simulink model "IdealGen_load_abc"  (R2023b)
settings: Solver=VariableStepAuto  StartTime=0.0  StopTime=Tend  RelTol=1e-3
undefined symbols (not defined in the file): C_hv_km, Cagg, f_nom, Ibase_hv, Ibase_lv, L_comp, L_grid, L_hv_km, l_t_ehvhv, l_t_hvmv, l_t_mvlv, Lagg, nWT, phase_shift_test_state, phase_shifts, PnomWT, R_grid, R_hv_km, r_t_ehvhv, r_t_hvmv, r_t_mvlv, Ragg, rocof_slope, Rocof_test_state, Sbase1, Sbase_t1, Trocof_end, Trocof_start, Ts_power, Vbase_ehv, Vbase_hv, Vbase_lv, Vbase_mv, voltage_sag_test_state
libraries: spsThreePhasePISectionLineLib x11, spsPower3phInstantaneousLib x5, spsControlledVoltageSourceLib x3, spsGroundLib x3, spsThreePhaseVIMeasurementLib x3, spsThreePhaseSeriesRLCBranchLib x3, spsThreePhaseTransformerTwoWindingsLib x3, spsdq0toabcLib x1, simulink x1, spsSampleandHoldLib x1, spsMultimeterLib x1, spsThreePhaseSeriesRLCLoadLib x1
settings Model: Creator=s183702  LastModifiedBy=Martin Pedersen

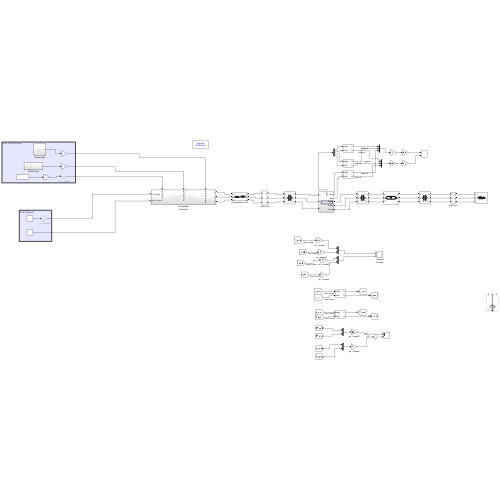
[thumbnail: Simulink's stored preview of the top-level diagram]
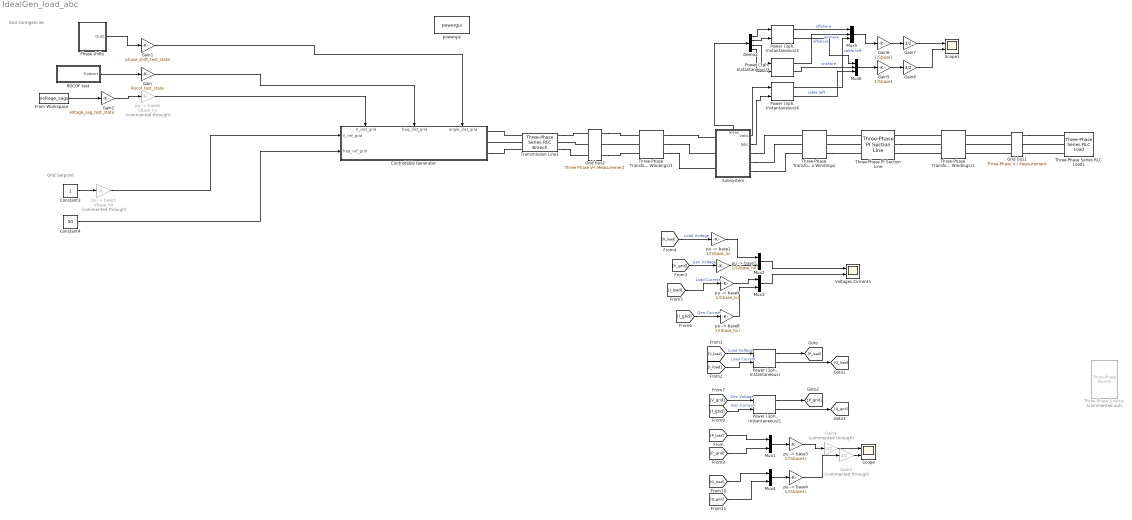
== system IdealGen_load_abc ==
  note: Grid Contigencies
  note: Grid Setpoint
  Constant3 : Constant
  Constant4 : Constant  Value=50
  Controllable Generator : Subsystem
      settings: PortSchema="{\"entries\":[{\"content\":{\"sides\":[{\"content\":{\"connectorIds\":[\"In1\",\"In2\"]},\"type\":\"ConnectorPlacement.EquallySpacedRectSide\",\"uuid\":\"c82e3ee4-47de-4631-9682-a189e406d2fd\"},{\"content\":{\"connectorIds\":[\"RConn1\",\"RConn2\",\"RConn3\"],\"side\":\"RIGHT\"},\"type\":\"ConnectorPlacement.EquallySpacedRectSide\",\"uuid\":\"b806e225-811d-4112-8c3d-45e9b8086e84\"},{\"content\":{\"connectorIds\":[\"In3\",\"In4\",\"In5\"],\"side\":\"TOP\"},\"type\":\"ConnectorPlacement.EquallySpacedRectSide\",\"uuid\":\"c79b677b-bc74-4454-b0f0-10f0f27e0767\"}]},\"type\":\"ConnectorPlacement.EquallySpacedConnector\",\"uuid\":\"44354c03-b4f0-403a-803b-b669dc1296a6\"}],\"packageUris\":[\"http://schema.mathworks.com/mf0/Connector/R2020b\"],\"version\":\"1.0\"}"
  Demux : Demux
  From Workspace : FromWorkspace  VariableName=voltage_sags
  Gain : Gain  Gain=Rocof_test_state
  Gain1 : Gain  Gain=phase_shift_test_state
  Gain2 : Gain  Gain=voltage_sag_test_state
  Gain3 : Gain  Commented=through  Gain=3/2
  Gain4 : Gain  Commented=through  Gain=3/2
  Gain5 : Gain  Gain=1/Sbase1
  Gain6 : Gain  Gain=1/Sbase1
  Gain7 : Gain  Gain=3/2
  Gain8 : Gain  Gain=3/2
  Grid bus1 : spsThreePhaseVIMeasurementLib/Three-Phase V-I Measurement  VoltageMeasurement=phase-to-phase  SetLabelV=on  LabelV=V_load  Vpu=off  VpuLL=off  CurrentMeasurement=yes  SetLabelI=on  LabelI=I_load  Ipu=off  Pbase=100e6  Vbase=500e3  OutputType=Complex  PhasorSimulation=off  PSBequivalent=0
  Grid bus2 : spsThreePhaseVIMeasurementLib/Three-Phase V-I Measurement  VoltageMeasurement=phase-to-phase  SetLabelV=on  LabelV=V_grid  Vpu=off  VpuLL=off  CurrentMeasurement=yes  SetLabelI=on  LabelI=I_grid  Ipu=off  Pbase=100e6  Vbase=500e3  OutputType=Complex  PhasorSimulation=off  PSBequivalent=0
  Mux{1..4} (4 alike) : Mux  Inputs=2
  Mux5 : Mux  Inputs=3
  Mux6 : Mux  Inputs=3
  Phase shifts : Subsystem
  Power (3ph, Instantaneous){,1..4} (5 alike) : spsPower3phInstantaneousLib/Power (3ph, Instantaneous)
  ROCOF test : Subsystem
  Scope : Scope  NumInputPorts=2
  Scope1 : Scope  NumInputPorts=2
  Subsystem : Subsystem
      settings: PortSchema="{\"entries\":[{\"content\":{\"sides\":[{\"content\":{\"connectorIds\":[\"LConn1\",\"LConn2\",\"LConn3\"]},\"type\":\"ConnectorPlacement.EquallySpacedRectSide\",\"uuid\":\"1e75b8ae-1ae2-41d3-b362-6bec791dcf00\"},{\"content\":{\"connectorIds\":[\"Out1\",\"Out2\",\"RConn1\",\"RConn2\",\"RConn3\"],\"side\":\"RIGHT\"},\"type\":\"ConnectorPlacement.EquallySpacedRectSide\",\"uuid\":\"b9649e6f-c713-4552-95ab-bed4ae3fc4ed\"},{\"content\":{\"connectorIds\":[\"Out3\"],\"side\":\"TOP\"},\"type\":\"ConnectorPlacement.EquallySpacedRectSide\",\"uuid\":\"245e241a-8feb-4dbf-8b97-336629a28915\"}]},\"type\":\"ConnectorPlacement.EquallySpacedConnector\",\"uuid\":\"8d181cc9-19cf-4cb2-b946-858b4ed04b70\"}],\"packageUris\":[\"http://schema.mathworks.com/mf0/Connector/R2020b\"],\"version\":\"1.0\"}"
  Three-Phase PI Section Line : spsThreePhasePISectionLineLib/Three-Phase PI Section Line  LConnTagsString=a|b|c  RConnTagsString=A|B|C  Length=1  Frequency=50  Resistances=[ 1 3]*Ragg  Inductances=[ 1 3]*Lagg  Capacitances=[ 1 0.6]*Cagg
  Three-Phase Series RLC Load1 : spsThreePhaseSeriesRLCLoadLib/Three-Phase Series RLC Load  LConnTagsString=A|B|C  Configuration=Y (grounded)  NominalVoltage=Vbase_lv*sqrt(3/2)  Vabc=[1e3 1e3 1e3]  Vabcp=[1e3 1e3 1e3]  NominalFrequency=f_nom  UnbalancedPower=off  ActivePower=PnomWT*nWT  InductivePower=0  CapacitivePower=0  Pabc=[10e3 9e3 11e3]  QLabc=[100 90 110]  QCabc=[100 90 110]  Pabcp=[10e3 9e3 11e3]  QLabcp=[100 90 110]  QCabcp=[100 90 110]  Measurements=None  LoadType=constant PQ
  Three-Phase Transformer (Two Windings) : spsThreePhaseTransformerTwoWindingsLib/Three-Phase Transformer (Two Windings)  Winding1Connection=Yg  Winding2Connection=Yg  CoreType=Three single-phase transformers  SetSaturation=off  Hysteresis=off  DataFile='hysteresis'  SetInitialFlux=off  Measurements=None  UNITS=pu  NominalPower=[ Sbase1 , f_nom ]  Winding1=[ Vbase_hv*sqrt(3/2) , r_t_hvmv/2 , l_t_hvmv/2]  Winding2=[ Vbase_mv*sqrt(3/2) , r_t_hvmv/2, l_t_hvmv/2 ]  Rm=500  Lm=500  L0=0.5  Saturation=[ 0,0 ; 0.0024,1.2 ; 1.0,1.52 ]  InitialFluxes=[ 0.8 , -0.8 , 0.7 ]  BreakLoop=off  DiscreteSolver=Trapezoidal iterative  DataType=off  TransfoNumber=1
  Three-Phase Transformer (Two Windings)1 : spsThreePhaseTransformerTwoWindingsLib/Three-Phase Transformer (Two Windings)  Winding1Connection=Yg  Winding2Connection=Yg  CoreType=Three single-phase transformers  SetSaturation=off  Hysteresis=off  DataFile='hysteresis'  SetInitialFlux=off  Measurements=None  UNITS=pu  NominalPower=[ Sbase_t1 , f_nom ]  Winding1=[ Vbase_mv*sqrt(3/2) , r_t_mvlv/2 , l_t_mvlv/2]  Winding2=[ Vbase_lv*sqrt(3/2) , r_t_mvlv/2, l_t_mvlv/2 ]  Rm=500  Lm=500  L0=0.5  Saturation=[ 0,0 ; 0.0024,1.2 ; 1.0,1.52 ]  InitialFluxes=[ 0.8 , -0.8 , 0.7 ]  BreakLoop=off  DiscreteSolver=Trapezoidal iterative  DataType=off  TransfoNumber=1
  Three-Phase Transformer (Two Windings)3 : spsThreePhaseTransformerTwoWindingsLib/Three-Phase Transformer (Two Windings)  Winding1Connection=Yg  Winding2Connection=Yg  CoreType=Three single-phase transformers  SetSaturation=off  Hysteresis=off  DataFile='hysteresis'  SetInitialFlux=off  Measurements=None  UNITS=pu  NominalPower=[ Sbase1*1.05, f_nom ]  Winding1=[ Vbase_ehv*sqrt(3/2) , r_t_ehvhv/2 , l_t_ehvhv/2]  Winding2=[ Vbase_hv*sqrt(3/2) ,r_t_ehvhv/2 , l_t_ehvhv/2 ]  Rm=500  Lm=500  L0=0.5  Saturation=[ 0,0 ; 0.0024,1.2 ; 1.0,1.52 ]  InitialFluxes=[ 0.8 , -0.8 , 0.7 ]  BreakLoop=off  DiscreteSolver=Trapezoidal iterative  DataType=off  TransfoNumber=1
  Three-Phase Source : spsThreePhaseSourceLib/Three-Phase Source  Commented=on  InternalConnection=Yg  VoltagePhases=off  Voltage=0.8*Vbase_lv*sqrt(3)/sqrt(2)  PhaseAngle=0  Voltage_phases=[25e3 25e3 25e3]/sqrt(3)  PhaseAngles_phases=[0 -120 +120]  Frequency=50  NonIdealSource=off  SpecifyImpedance=off  Resistance=0.8929  Inductance=16.58e-3  ShortCircuitLevel=100e6  BaseVoltage=25e3  XRratio=7  BusType=swing  Pref=10e3  Qref=0  Prefabc=[10e3, 10e3, 10e3]  Qrefabc=[0, 0, 0]  Qmin=-inf  Qmax=inf
  Transmission Line1 : spsThreePhaseSeriesRLCBranchLib/Three-Phase Series RLC Branch  LConnTagsString=A|B|C  RConnTagsString=A|B|C  BranchType=RL  Resistance=R_grid  Inductance=L_grid  Capacitance=0  Measurements=None
  Voltages Currents : Scope  NumInputPorts=2
  powergui : spspowerguiLib/powergui  Priority=1  SimulationMode=Discrete  SampleTime=Ts_power  frequency=60  Iterations=50  frequencyindice=50  Pbase=100e6  ErrMax=1e-4  UnitsV=kV  UnitsW=MW  buscounter=0  FunctionMessages=off  echomessages=off  EnableUseOfTLC=off  CurrentSourceSwitches=off  DisableSnubberDevices=off  DisableRonSwitches=off  DisableVfSwitches=off  DisplayEquations=off  AutomaticDiscreteSolvers=off  SolverType=Tustin/Backward Euler (TBE)  Interpol=off  ExternalGateDelay=off  methode=off  Ts=100  x0status=blocks  SPID=on  SwTol=0  HookPort=off  NonlinearTolerance=1e-4  nMaxIteration=100  ContinueOnMaxIteration=off  RestoreLinks=warning  ResistiveCurrentMeasurement=off  Frange=[0:2:500]  Ylog=off  Xlog=on  ShowGrid=off  save=off  variable=ZData  structure=0  ZoomFFT=off  StartTime=0.0  cycles=1  DisplayStyle=1  fundamental=60  FreqAxis=off  MaxFrequency=1000  frequencyindicesteady=1  RmsSteady=1  display=off
  "pu -> base1" : Gain  Gain=1/(Vbase_lv)
  "pu -> base3" : Gain  Gain=1/(Sbase1)
  "pu -> base4" : Gain  Gain=1/(Sbase1)
  "pu -> base5" : Gain  Commented=through  Gain=Vbase_hv
  "pu -> base6" : Gain  Commented=through  Gain=Vbase_hv
  "pu -> base7" : Gain  Gain=1/(Vbase_hv)
  "pu -> base8" : Gain  Gain=1/(Ibase_hv)
  "pu -> base9" : Gain  Gain=1/(Ibase_lv)
  wires:
  [I_load] -> "pu -> base9"/1  "Load Current"
  [V_load] -> "pu -> base1"/1  "Load Voltage"
  [V_grid] -> "pu -> base7"/1  "Gen Voltage"
  [I_grid] -> "pu -> base8"/1  "Gen Current"
  Mux3/1 -> Voltages Currents/2
  "pu -> base5"/1 -> Controllable Generator/1(V_ref_grid)
  Constant4/1 -> Controllable Generator/2(freq_ref_grid)
  Gain/1 -> Controllable Generator/4(freq_dist_grid)
  Gain1/1 -> Controllable Generator/5(angle_dist_grid)
  [V_load] -> "Power (3ph, Instantaneous)"/1  "Load Voltage"
  [I_load] -> "Power (3ph, Instantaneous)"/2  "Load Current"
  [V_grid] -> "Power (3ph, Instantaneous)1"/1  "Gen Voltage"
  [I_grid] -> "Power (3ph, Instantaneous)1"/2  "Gen Current"
  "Power (3ph, Instantaneous)"/1 -> [P_load]
  "Power (3ph, Instantaneous)"/2 -> [Q_load]
  "Power (3ph, Instantaneous)1"/1 -> [P_grid]
  "Power (3ph, Instantaneous)1"/2 -> [Q_grid]
  [Q_load] -> Mux4/1
  [Q_grid] -> Mux4/2
  [P_grid] -> Mux1/2
  [P_load] -> Mux1/1
  Mux4/1 -> "pu -> base4"/1
  Mux1/1 -> "pu -> base3"/1
  "pu -> base3"/1 -> Gain4/1
  "pu -> base4"/1 -> Gain3/1
  Constant3/1 -> "pu -> base5"/1
  Phase shifts/1(Out2) -> Gain1/1
  From Workspace/1 -> Gain2/1
  ROCOF test/1(Outport) -> Gain/1
  "pu -> base6"/1 -> Controllable Generator/3(V_dist_grid)
  Gain2/1 -> "pu -> base6"/1
  Mux2/1 -> Voltages Currents/1
  "pu -> base1"/1 -> Mux2/1
  "pu -> base7"/1 -> Mux2/2
  "pu -> base8"/1 -> Mux3/2
  "pu -> base9"/1 -> Mux3/1
  Gain3/1 -> Scope/2
  Gain4/1 -> Scope/1
  "Power (3ph, Instantaneous)3"/1 -> Mux5/2  "onshore"
  Demux/3 -> "Power (3ph, Instantaneous)3"/1
  Demux/2 -> "Power (3ph, Instantaneous)2"/2
  Subsystem/3(meas) -> Demux/1
  "Power (3ph, Instantaneous)2"/1 -> Mux5/1  "offshore"
  "Power (3ph, Instantaneous)3"/2 -> Mux6/2  "onshore"
  Demux/4 -> "Power (3ph, Instantaneous)3"/2
  "Power (3ph, Instantaneous)2"/2 -> Mux6/1  "offshore"
  Demux/1 -> "Power (3ph, Instantaneous)2"/1
  "Power (3ph, Instantaneous)4"/1 -> Mux5/3  "cable left"
  "Power (3ph, Instantaneous)4"/2 -> Mux6/3  "cable left"
  Mux5/1 -> Gain6/1
  Mux6/1 -> Gain5/1
  Gain6/1 -> Gain7/1
  Gain5/1 -> Gain8/1
  Gain7/1 -> Scope1/1
  Gain8/1 -> Scope1/2
  Subsystem/1(Vabc) -> "Power (3ph, Instantaneous)4"/1
  Subsystem/2(Iabc) -> "Power (3ph, Instantaneous)4"/2
  connections:
  Three-Phase Transformer (Two Windings)1/LConn1 -- Three-Phase PI Section Line/RConn1
  Grid bus1/RConn1 -- Three-Phase Series RLC Load1/LConn1
  Three-Phase Series RLC Load1/LConn2 -- Grid bus1/RConn2
  Grid bus1/RConn3 -- Three-Phase Series RLC Load1/LConn3
  Transmission Line1/RConn1 -- Grid bus2/LConn1
  Grid bus2/LConn2 -- Transmission Line1/RConn2
  Transmission Line1/RConn3 -- Grid bus2/LConn3
  Transmission Line1/LConn1 -- Controllable Generator/RConn1
  Transmission Line1/LConn2 -- Controllable Generator/RConn2
  Controllable Generator/RConn3 -- Transmission Line1/LConn3
  Three-Phase PI Section Line/LConn2 -- Three-Phase Transformer (Two Windings)/RConn2
  Three-Phase PI Section Line/LConn1 -- Three-Phase Transformer (Two Windings)/RConn1
  Three-Phase Transformer (Two Windings)/RConn3 -- Three-Phase PI Section Line/LConn3
  Three-Phase PI Section Line/RConn2 -- Three-Phase Transformer (Two Windings)1/LConn2
  Three-Phase Transformer (Two Windings)1/LConn3 -- Three-Phase PI Section Line/RConn3
  Grid bus1/LConn1 -- Three-Phase Transformer (Two Windings)1/RConn1
  Grid bus1/LConn2 -- Three-Phase Transformer (Two Windings)1/RConn2
  Grid bus1/LConn3 -- Three-Phase Transformer (Two Windings)1/RConn3
  Three-Phase Transformer (Two Windings)3/LConn2 -- Grid bus2/RConn2
  Grid bus2/RConn1 -- Three-Phase Transformer (Two Windings)3/LConn1
  Grid bus2/RConn3 -- Three-Phase Transformer (Two Windings)3/LConn3
  Three-Phase Transformer (Two Windings)3/RConn1 -- Subsystem/LConn1
  Subsystem/RConn1 -- Three-Phase Transformer (Two Windings)/LConn1
  Three-Phase Transformer (Two Windings)3/RConn2 -- Subsystem/LConn2
  Subsystem/RConn2 -- Three-Phase Transformer (Two Windings)/LConn2
  Three-Phase Transformer (Two Windings)3/RConn3 -- Subsystem/LConn3
  Subsystem/RConn3 -- Three-Phase Transformer (Two Windings)/LConn3

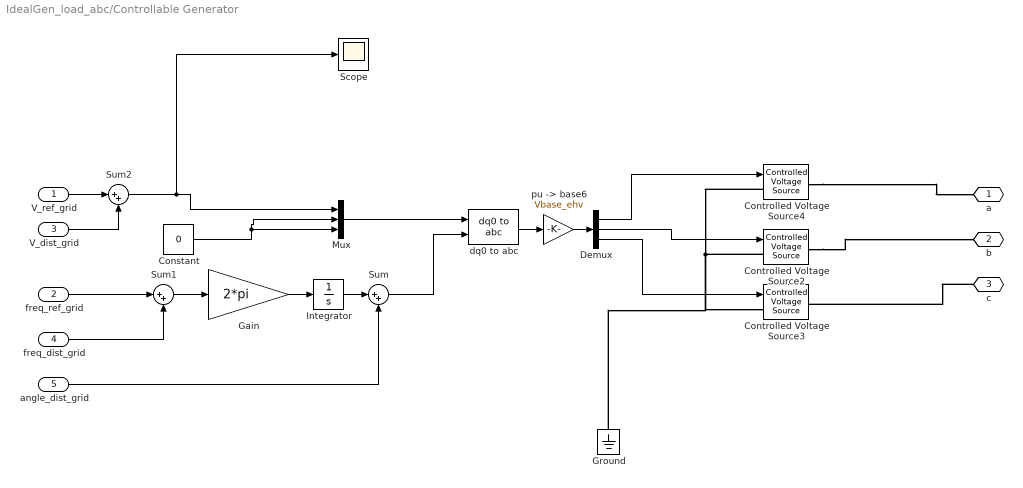
== system IdealGen_load_abc/Controllable Generator ==
  V_ref_grid : Inport
  freq_ref_grid : Inport  Port=2
  V_dist_grid : Inport  Port=3
  freq_dist_grid : Inport  Port=4
  angle_dist_grid : Inport  Port=5
  Constant : Constant  Value=0
  Controlled Voltage Source2 : spsControlledVoltageSourceLib/Controlled Voltage Source  Initialize=on  Source_Type=AC  Amplitude=Vbase_hv  Phase=-120  Frequency=50  Measurements=None
  Controlled Voltage Source3 : spsControlledVoltageSourceLib/Controlled Voltage Source  Initialize=on  Source_Type=AC  Amplitude=Vbase_hv  Phase=120  Frequency=50  Measurements=None
  Controlled Voltage Source4 : spsControlledVoltageSourceLib/Controlled Voltage Source  Initialize=on  Source_Type=AC  Amplitude=Vbase_hv  Phase=0  Frequency=50  Measurements=None
  Demux : Demux  Outputs=3
  Gain : Gain  Gain=2*pi
  Ground : spsGroundLib/Ground  LConnTagsString=a
  Integrator : Integrator
  Mux : Mux  Inputs=3
  Scope : Scope
  Sum : Sum  Inputs=|++
  Sum1 : Sum  Inputs=|++
  Sum2 : Sum  Inputs=|++
  dq0 to abc : spsdq0toabcLib/dq0 to abc  Alignment=90 degrees behind phase A axis
  "pu -> base6" : Gain  Gain=Vbase_ehv
  a : PMIOPort  Side=Right
  b : PMIOPort  Port=2  Side=Right
  c : PMIOPort  Port=3  Side=Right
  wires:
  Demux/1 -> Controlled Voltage Source4/1
  Demux/2 -> Controlled Voltage Source2/1
  Demux/3 -> Controlled Voltage Source3/1
  Mux/1 -> dq0 to abc/1
  Constant/1 -> Mux/2, Mux/3
  dq0 to abc/1 -> "pu -> base6"/1
  Sum2/1 -> Scope/1, Mux/1
  Gain/1 -> Integrator/1
  Integrator/1 -> Sum/1
  angle_dist_grid/1 -> Sum/2
  freq_dist_grid/1 -> Sum1/2
  Sum1/1 -> Gain/1
  freq_ref_grid/1 -> Sum1/1
  Sum/1 -> dq0 to abc/2
  V_ref_grid/1 -> Sum2/1
  V_dist_grid/1 -> Sum2/2
  "pu -> base6"/1 -> Demux/1
  connections:
  Controlled Voltage Source2/LConn1 -- Controlled Voltage Source4/LConn1 -- Ground/LConn1 -- Controlled Voltage Source3/LConn1
  c/RConn1 -- Controlled Voltage Source3/RConn1
  Controlled Voltage Source4/RConn1 -- a/RConn1
  Controlled Voltage Source2/RConn1 -- b/RConn1

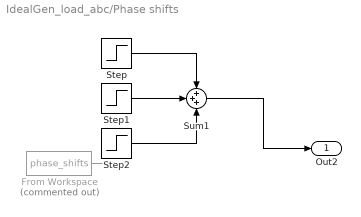
== system IdealGen_load_abc/Phase shifts ==
  From Workspace : FromWorkspace  Commented=on  VariableName=phase_shifts  OutputAfterFinalValue=Setting to zero
  Step : Step  Time=phase_shifts(1,1)  After=phase_shifts(1,2)  SampleTime=0
  Step1 : Step  Time=phase_shifts(2,1)  After=phase_shifts(2,2)  SampleTime=0
  Step2 : Step  Time=phase_shifts(3,1)  After=phase_shifts(3,2)  SampleTime=0
  Sum1 : Sum  Inputs=+++
  Out2 : Outport
  wires:
  Sum1/1 -> Out2/1
  Step/1 -> Sum1/1
  Step2/1 -> Sum1/3
  From Workspace/1 -> ?
  Step1/1 -> Sum1/2

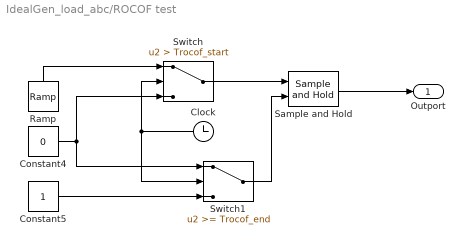
== system IdealGen_load_abc/ROCOF test ==
  Clock : Clock
  Constant4 : Constant  Value=0
  Constant5 : Constant
  Ramp : simulink/Sources/Ramp  slope=rocof_slope  start=Trocof_start  InitialOutput=0
  Sample and Hold : spsSampleandHoldLib/Sample and Hold  ic=0  Ts=0
      settings: LibrarySourceBlock=|
      | sps_lib/Control/Sample and
      | Hold
  Switch : Switch  Criteria=u2 > Threshold  Threshold=Trocof_start  SaturateOnIntegerOverflow=off  InputSameDT=off
  Switch1 : Switch  Threshold=Trocof_end  SaturateOnIntegerOverflow=off  InputSameDT=off
  Outport : Outport
  wires:
  Clock/1 -> Switch/2, Switch1/2
  Constant4/1 -> Switch/3, Switch1/1
  Sample and Hold/1 -> Outport/1
  Ramp/1 -> Switch/1
  Constant5/1 -> Switch1/3
  Switch/1 -> Sample and Hold/1
  Switch1/1 -> Sample and Hold/2

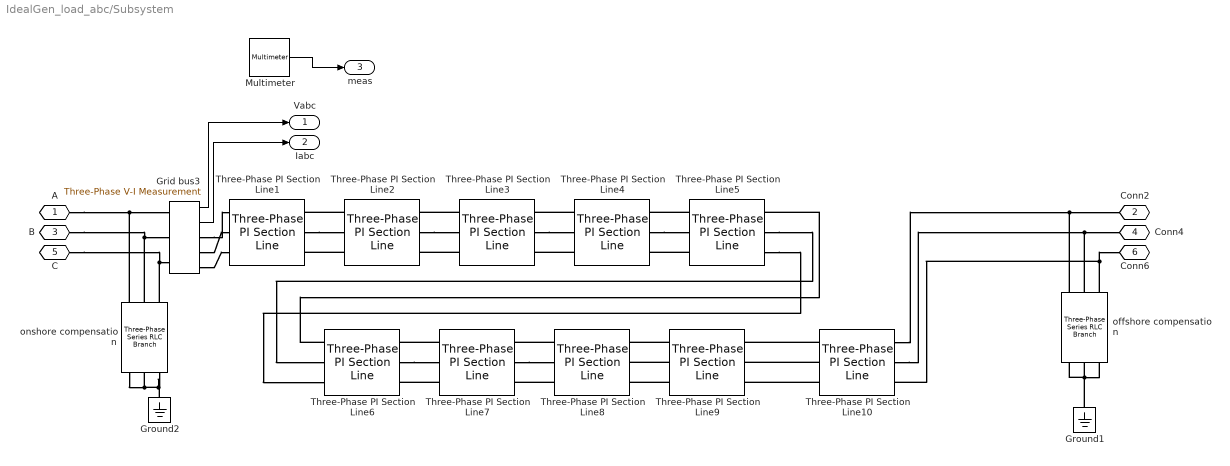
== system IdealGen_load_abc/Subsystem ==
  Grid bus3 : spsThreePhaseVIMeasurementLib/Three-Phase V-I Measurement  VoltageMeasurement=phase-to-ground  SetLabelV=off  LabelV=V_grid  Vpu=off  VpuLL=off  CurrentMeasurement=yes  SetLabelI=off  LabelI=I_grid  Ipu=off  Pbase=100e6  Vbase=500e3  OutputType=Complex  PhasorSimulation=off  PSBequivalent=0
  Ground1 : spsGroundLib/Ground  LConnTagsString=a
  Ground2 : spsGroundLib/Ground  LConnTagsString=a
  Multimeter : spsMultimeterLib/Multimeter  L=12  sel=[1 2 3 7 8 9 4 5 6 10 11 12]  yselected={}  Gain=[1 1 1 1 1 1 1 1 1 1 1 1]  OutputType=Complex  PlotAtSimulationStop=off  PhasorSimulation=off
  Three-Phase PI Section Line{1..10} (10 alike) : spsThreePhasePISectionLineLib/Three-Phase PI Section Line  LConnTagsString=a|b|c  RConnTagsString=A|B|C  Length=100/10  Frequency=50  Resistances=[ 1 3]*R_hv_km  Inductances=[ 1 3]*L_hv_km  Capacitances=[ 1 0.6]*C_hv_km
  offshore compensation : spsThreePhaseSeriesRLCBranchLib/Three-Phase Series RLC Branch  LConnTagsString=A|B|C  RConnTagsString=A|B|C  BranchType=L  Resistance=7.648620605468750  Inductance=L_comp  Capacitance=1e-6  Measurements=Branch voltages and currents
  onshore compensation : spsThreePhaseSeriesRLCBranchLib/Three-Phase Series RLC Branch  LConnTagsString=A|B|C  RConnTagsString=A|B|C  BranchType=L  Resistance=7.648620605468750  Inductance=L_comp  Capacitance=1e-6  Measurements=Branch voltages and currents
  A : PMIOPort  Side=Left
  Conn2 : PMIOPort  Port=2  Side=Right
  B : PMIOPort  Port=3  Side=Left
  Conn4 : PMIOPort  Port=4  Side=Right
  C : PMIOPort  Port=5  Side=Left
  Conn6 : PMIOPort  Port=6  Side=Right
  Vabc : Outport
  Iabc : Outport  Port=2
  meas : Outport  Port=3
  wires:
  Grid bus3/1 -> Vabc/1
  Grid bus3/2 -> Iabc/1
  Multimeter/1 -> meas/1
  connections:
  offshore compensation/LConn2 -- Conn4/RConn1 -- Three-Phase PI Section Line10/RConn2
  offshore compensation/LConn1 -- Three-Phase PI Section Line10/RConn1 -- Conn2/RConn1
  Ground2/LConn1 -- onshore compensation/RConn3 -- onshore compensation/RConn1 -- onshore compensation/RConn2
  onshore compensation/LConn3 -- C/RConn1 -- Grid bus3/LConn3
  Ground1/LConn1 -- offshore compensation/RConn1 -- offshore compensation/RConn3 -- offshore compensation/RConn2
  offshore compensation/LConn3 -- Conn6/RConn1 -- Three-Phase PI Section Line10/RConn3
  onshore compensation/LConn1 -- A/RConn1 -- Grid bus3/LConn1
  onshore compensation/LConn2 -- B/RConn1 -- Grid bus3/LConn2
  Grid bus3/RConn1 -- Three-Phase PI Section Line1/LConn1
  Grid bus3/RConn3 -- Three-Phase PI Section Line1/LConn3
  Grid bus3/RConn2 -- Three-Phase PI Section Line1/LConn2
  Three-Phase PI Section Line9/LConn1 -- Three-Phase PI Section Line8/RConn1
  Three-Phase PI Section Line9/LConn2 -- Three-Phase PI Section Line8/RConn2
  Three-Phase PI Section Line9/LConn3 -- Three-Phase PI Section Line8/RConn3
  Three-Phase PI Section Line10/LConn2 -- Three-Phase PI Section Line9/RConn2
  Three-Phase PI Section Line10/LConn1 -- Three-Phase PI Section Line9/RConn1
  Three-Phase PI Section Line10/LConn3 -- Three-Phase PI Section Line9/RConn3
  Three-Phase PI Section Line8/LConn1 -- Three-Phase PI Section Line7/RConn1
  Three-Phase PI Section Line7/RConn2 -- Three-Phase PI Section Line8/LConn2
  Three-Phase PI Section Line8/LConn3 -- Three-Phase PI Section Line7/RConn3
  Three-Phase PI Section Line7/LConn1 -- Three-Phase PI Section Line6/RConn1
  Three-Phase PI Section Line6/RConn2 -- Three-Phase PI Section Line7/LConn2
  Three-Phase PI Section Line7/LConn3 -- Three-Phase PI Section Line6/RConn3
  Three-Phase PI Section Line6/LConn1 -- Three-Phase PI Section Line5/RConn1
  Three-Phase PI Section Line5/RConn2 -- Three-Phase PI Section Line6/LConn2
  Three-Phase PI Section Line5/RConn3 -- Three-Phase PI Section Line6/LConn3
  Three-Phase PI Section Line5/LConn1 -- Three-Phase PI Section Line4/RConn1
  Three-Phase PI Section Line4/RConn2 -- Three-Phase PI Section Line5/LConn2
  Three-Phase PI Section Line5/LConn3 -- Three-Phase PI Section Line4/RConn3
  Three-Phase PI Section Line4/LConn1 -- Three-Phase PI Section Line3/RConn1
  Three-Phase PI Section Line3/RConn2 -- Three-Phase PI Section Line4/LConn2
  Three-Phase PI Section Line4/LConn3 -- Three-Phase PI Section Line3/RConn3
  Three-Phase PI Section Line3/LConn1 -- Three-Phase PI Section Line2/RConn1
  Three-Phase PI Section Line2/RConn2 -- Three-Phase PI Section Line3/LConn2
  Three-Phase PI Section Line3/LConn3 -- Three-Phase PI Section Line2/RConn3
  Three-Phase PI Section Line2/LConn1 -- Three-Phase PI Section Line1/RConn1
  Three-Phase PI Section Line1/RConn2 -- Three-Phase PI Section Line2/LConn2
  Three-Phase PI Section Line2/LConn3 -- Three-Phase PI Section Line1/RConn3
